simulink model "Zoom"  (R2025b)
settings: Solver=VariableStepAuto  StartTime=0.0  StopTime=0.1  RelTol=1e-3
undefined symbols (not defined in the file): designMultirateFIR, dspblkCoreblockFVToolHelper, gcbh, NBits
libraries: dspmlti4 x4, dspsigops x2, simulink_extras x1, msbAdcArchitectures x1
settings Model: Creator=sohom  LastModifiedBy=sohom

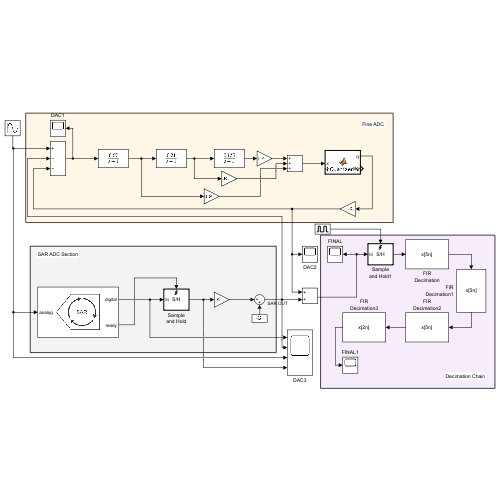
[thumbnail: Simulink's stored preview of the top-level diagram]
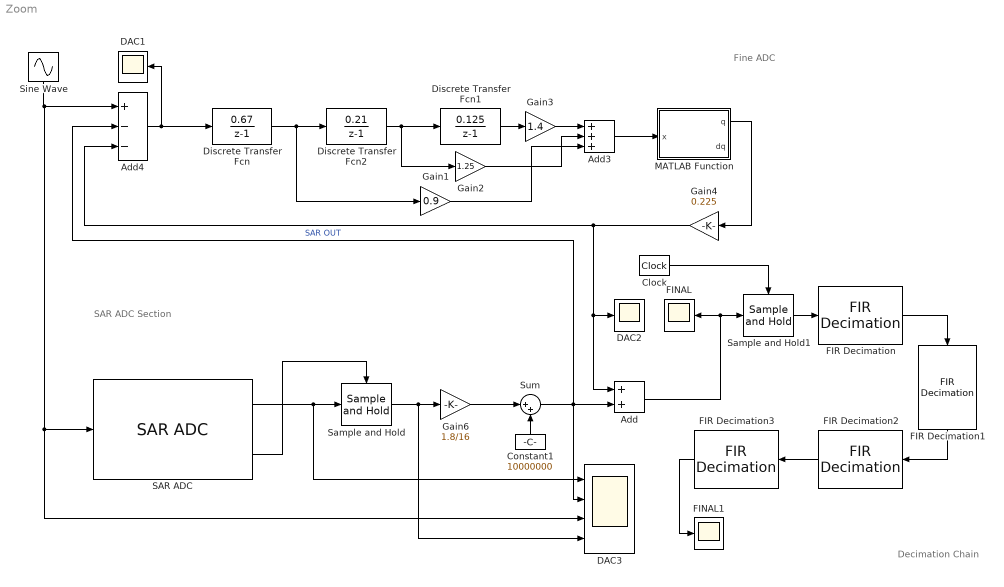
== system Zoom ==
  note: Fine ADC
  note: Decimation Chain
  note: SAR ADC Section
  Add : Sum
  Add3 : Sum  Inputs=+++
  Add4 : Sum  Inputs=+--
  Clock : simulink_extras/Flip Flops/Clock  period=1e-6
  Constant1 : Constant  Value=10000000
  DAC1 : Scope
      settings: ActiveDisplayYMinimum=-0.20794044337957318  ActiveDisplayYMaximum=0.16691914128015831
  DAC2 : Scope
      settings: ActiveDisplayYMinimum=-0.140625  ActiveDisplayYMaximum=0.140625  DataLoggingVariableName=ScopeData2
  DAC3 : Scope  NumInputPorts=4
      settings: ActiveDisplayYMinimum=1.4002266972206661  ActiveDisplayYMaximum=1.5420146284485854  DataLoggingVariableName=ScopeData3
  Discrete Transfer Fcn : DiscreteTransferFcn  LoadFcn=dspblkCoreblockFVToolHelper(gcbh,'load');  Numerator=[0.67]  Denominator=[1 -1]
      settings: CopyFcn=dspblkCoreblockFVToolHelper(gcbh,'copy');  DeleteFcn=dspblkCoreblockFVToolHelper(gcbh,'close');  ModelCloseFcn=dspblkCoreblockFVToolHelper(gcbh,'close');  PreSaveFcn=dspblkCoreblockFVToolHelper(gcbh,'presave');  PostSaveFcn=dspblkCoreblockFVToolHelper(gcbh,'postsave');  CloseFcn=dspblkCoreblockFVToolHelper(gcbh,'close');
  Discrete Transfer Fcn1 : DiscreteTransferFcn  LoadFcn=dspblkCoreblockFVToolHelper(gcbh,'load');  Numerator=[0.125]  Denominator=[1 -1]
      settings: CopyFcn=dspblkCoreblockFVToolHelper(gcbh,'copy');  DeleteFcn=dspblkCoreblockFVToolHelper(gcbh,'close');  ModelCloseFcn=dspblkCoreblockFVToolHelper(gcbh,'close');  PreSaveFcn=dspblkCoreblockFVToolHelper(gcbh,'presave');  PostSaveFcn=dspblkCoreblockFVToolHelper(gcbh,'postsave');  CloseFcn=dspblkCoreblockFVToolHelper(gcbh,'close');
  Discrete Transfer Fcn2 : DiscreteTransferFcn  LoadFcn=dspblkCoreblockFVToolHelper(gcbh,'load');  Numerator=[0.21]  Denominator=[1 -1]
      settings: CopyFcn=dspblkCoreblockFVToolHelper(gcbh,'copy');  DeleteFcn=dspblkCoreblockFVToolHelper(gcbh,'close');  ModelCloseFcn=dspblkCoreblockFVToolHelper(gcbh,'close');  PreSaveFcn=dspblkCoreblockFVToolHelper(gcbh,'presave');  PostSaveFcn=dspblkCoreblockFVToolHelper(gcbh,'postsave');  CloseFcn=dspblkCoreblockFVToolHelper(gcbh,'close');
  FINAL : Scope
      settings: ActiveDisplayYMinimum=-2.172928125  ActiveDisplayYMaximum=2.0653531249999997
  FINAL1 : Scope
      settings: ActiveDisplayYMinimum=-0.390480159683964  ActiveDisplayYMaximum=0.627797741111165  DataLoggingVariableName=ScopeData4
  FIR Decimation : dspmlti4/FIR Decimation  FilterSource=Auto  h=designMultirateFIR(1,2)  D=5  filtStruct=Direct form  FilterObject=FDECIM  framing=Allow multirate processing  AllowArbitraryInputLength=off  inputOffset=0  outputBufInitCond=0  roundingMode=Floor  overflowMode=off  firstCoeffDataTypeStr=Inherit: Same word length as input  firstCoeffMin=[]  firstCoeffMax=[]  firstCoeffLastDataTypeStr=Inherit: Same word length as input  outputDataTypeStr=Inherit: Same as accumulator  outputMin=[]  outputMax=[]  outputLastDataTypeStr=Inherit: Same as accumulator
      settings: LibrarySourceBlock=|
      | dsphdlsupportfiltering/FIR
      | Decimation
  FIR Decimation1 : dspmlti4/FIR Decimation  FilterSource=Auto  h=designMultirateFIR(1,2)  D=5  filtStruct=Direct form  FilterObject=FDECIM  framing=Allow multirate processing  AllowArbitraryInputLength=off  inputOffset=0  outputBufInitCond=0  roundingMode=Floor  overflowMode=off  firstCoeffDataTypeStr=Inherit: Same word length as input  firstCoeffMin=[]  firstCoeffMax=[]  firstCoeffLastDataTypeStr=Inherit: Same word length as input  outputDataTypeStr=Inherit: Same as accumulator  outputMin=[]  outputMax=[]  outputLastDataTypeStr=Inherit: Same as accumulator
      settings: LibrarySourceBlock=|
      | dsphdlsupportfiltering/FIR
      | Decimation
  FIR Decimation2 : dspmlti4/FIR Decimation  FilterSource=Auto  h=designMultirateFIR(1,2)  D=5  filtStruct=Direct form  FilterObject=FDECIM  framing=Allow multirate processing  AllowArbitraryInputLength=off  inputOffset=0  outputBufInitCond=0  roundingMode=Floor  overflowMode=off  firstCoeffDataTypeStr=Inherit: Same word length as input  firstCoeffMin=[]  firstCoeffMax=[]  firstCoeffLastDataTypeStr=Inherit: Same word length as input  outputDataTypeStr=Inherit: Same as accumulator  outputMin=[]  outputMax=[]  outputLastDataTypeStr=Inherit: Same as accumulator
      settings: LibrarySourceBlock=|
      | dsphdlsupportfiltering/FIR
      | Decimation
  FIR Decimation3 : dspmlti4/FIR Decimation  FilterSource=Auto  h=designMultirateFIR(1,2)  D=2  filtStruct=Direct form  FilterObject=FDECIM  framing=Allow multirate processing  AllowArbitraryInputLength=off  inputOffset=0  outputBufInitCond=0  roundingMode=Floor  overflowMode=off  firstCoeffDataTypeStr=Inherit: Same word length as input  firstCoeffMin=[]  firstCoeffMax=[]  firstCoeffLastDataTypeStr=Inherit: Same word length as input  outputDataTypeStr=Inherit: Same as accumulator  outputMin=[]  outputMax=[]  outputLastDataTypeStr=Inherit: Same as accumulator
      settings: LibrarySourceBlock=|
      | dsphdlsupportfiltering/FIR
      | Decimation
  Gain1 : Gain  Gain=0.9
  Gain2 : Gain  Gain=1.25
  Gain3 : Gain  Gain=1.4
  Gain4 : Gain  Gain=0.225
  Gain6 : Gain  Gain=1.8/16
  MATLAB Function : MATLAB Function  TreatAsAtomicUnit=on
  SAR ADC : msbAdcArchitectures/SAR ADC  DACVoltages=[-5:5]  DACINLVoltages=tanh([-5:5])  NBits=5  InputRange=[-1.8 1.8]  ExtStartClk=off  StartFreq=2e4  StartClkJitter=0  SARFreq=2e5  MatchScale=off  OutputPolarity=Auto  OutDataType=fixdt(1,NBits)  EnableLinearityImpairments=off  OffsetError=1  OffsetErrorUnit=LSB  GainError=2  GainErrorUnit=LSB
  Sample and Hold : dspsigops/Sample and Hold  trig=Rising edge  initCond=0  latchinput=off
  Sample and Hold1 : dspsigops/Sample and Hold  trig=Rising edge  initCond=0  latchinput=off
  Sine Wave : Sin  Amplitude=1.8  Frequency=1000  SampleTime=0
  Sum : Sum  Inputs=|++
  wires:
  Add4/1 -> Discrete Transfer Fcn/1, DAC1/1
  Discrete Transfer Fcn2/1 -> Gain2/1, Discrete Transfer Fcn1/1
  Discrete Transfer Fcn/1 -> Gain1/1, Discrete Transfer Fcn2/1
  Discrete Transfer Fcn1/1 -> Gain3/1
  Gain3/1 -> Add3/1
  Gain2/1 -> Add3/2
  Gain1/1 -> Add3/3
  Gain4/1 -> DAC2/1, Add/1, Add4/3
  Add/1 -> Sample and Hold1/1, FINAL/1
  Gain6/1 -> Sum/1
  Constant1/1 -> Sum/2
  SAR ADC/1 -> DAC3/1, Sample and Hold/1
  Sample and Hold/1 -> DAC3/4, Gain6/1
  SAR ADC/2 -> Sample and Hold/Trigger
  Sum/1 -> Add/2, Add4/2, DAC3/2  "SAR OUT"
  Add3/1 -> MATLAB Function/1(x)
  MATLAB Function/1(q) -> Gain4/1
  Sine Wave/1 -> Add4/1, DAC3/3, SAR ADC/1
  Sample and Hold1/1 -> FIR Decimation/1
  Clock/1 -> Sample and Hold1/Trigger
  FIR Decimation/1 -> FIR Decimation1/1
  FIR Decimation1/1 -> FIR Decimation2/1
  FIR Decimation2/1 -> FIR Decimation3/1
  FIR Decimation3/1 -> FINAL1/1

== matlab function Zoom/MATLAB Function ==
  data: x input; q output; dq output
function [q, dq] = bitQuantizer1bit(x)
if x >= 0
    q = 1;
else
    q = -1;
end
dq = q;
